simulink model "Aerogen2019NoActuator"  (R2019b)
settings: Solver=FixedStepAuto  StartTime=0.0  StopTime=10  FixedStep=0.001  RelTol=1e-6  EnableMultiTasking=on
values from neighbouring files (symbols this model uses):
  Bm = 0.001    [Trim_Lin.m]    (also in controlExercise.m)
  c1 = 0.51763    [Trim_Lin.m]    (also in controlExercise.m)
  c2 = 116    [Trim_Lin.m]    (also in controlExercise.m)
  c3 = 0.4    [Trim_Lin.m]    (also in controlExercise.m)
  c4 = 5    [Trim_Lin.m]    (also in controlExercise.m)
  c5 = 21    [Trim_Lin.m]    (also in controlExercise.m)
  c6 = 0.006795    [Trim_Lin.m]    (also in controlExercise.m)
  J = 10    [Trim_Lin.m]    (also in controlExercise.m = 0.1)
  Ke = 1.3717    [Trim_Lin.m]    (also in controlExercise.m)
  La = 0.028    [Trim_Lin.m]    (also in controlExercise.m)
  R = 10    [Trim_Lin.m]    (also in controlExercise.m)
  Ra = 2.58    [Trim_Lin.m]    (also in controlExercise.m)
  Rho = 1.225    [Trim_Lin.m]    (also in controlExercise.m)
  Rpala = 1.6    [Trim_Lin.m]    (also in controlExercise.m)
  Tf = 0.1    [Trim_Lin.m]    (also in controlExercise.m)
  Vw = 10    [Trim_Lin.m]    (also in controlExercise.m)
settings Model: ExtModeTrigDuration=100  Creator=Ignacio  LastModifiedBy=Carlos
settings SolverCC: PositivePriorityOrder=on
settings DataIOCC: LimitDataPoints=on  SaveFormat=Array  ReturnWorkspaceOutputs=off
settings OptimizationCC: DefaultParameterBehavior=Inlined  LifeSpan=1  MaxStackSize=64  EfficientTunableParamExpr=on
settings DebuggingCC: UnderspecifiedInitializationDetection=Classic  MergeDetectMultiDrivingBlocksExec=none  AllowSymbolicDim=off  SFUnexpectedBacktrackingDiag=warning  SFNoUnconditionalDefaultTransitionDiag=warning  SFExecutionAtInitializationDiag=none  ArithmeticOperatorsInVariantConditions=warning
settings HardwareCC: ProdBitPerPointer=32  ProdBitPerSizeT=32  ProdBitPerPtrDiffT=32  ProdLargestAtomicInteger=Long  ProdLargestAtomicFloat=Double  ProdWordSize=32  ProdHWDeviceType=ARM Compatible->ARM Cortex
settings ModelReferenceCC: PropagateSignalLabelsOutOfModel=off
settings SFSimCC: SimUseLocalCustomCode=off  MATLABDynamicMemAlloc=off  CustomCodeUndefinedFunction=UseInterfaceOnly
settings RTWCC: SystemTargetFile=ert.tlc  TemplateMakefile=ert_default_tmf  GenerateReport=on  RTWVerbose=off  RTWUseLocalCustomCode=off  Toolchain=GNU GCC Raspberry Pi  IncludeHyperlinkInReport=on  LaunchReport=on  GenerateTraceInfo=on  GenerateTraceReport=on  GenerateTraceReportSl=on  GenerateTraceReportSf=on  GenerateTraceReportEml=on
settings CodeAppCC: ForceParamTrailComments=on  IgnoreCustomStorageClasses=off  OperatorAnnotations=on  SimulinkDataObjDesc=on  SFDataObjDesc=on  MATLABFcnDesc=on  InsertBlockDesc=on  StateflowObjectComments=on  MATLABSourceComments=on
settings ERTTargetCC: MultiwordLength=2048  SupportVariableSizeSignals=on  ERTCustomFileTemplate=example_file_process.tlc
settings ConfigComp: CovMetricSettings=dw  CovHTMLOptions=-sRT=1 -aTS=1 -bRG=1 -bTC=1 -hTR=0 -nFC=0 -scm=1 -bcm=1 -xEv=0  CovHtmlReporting=on  CovSaveCumulativeToWorkspaceVar=on  CovSaveSingleToWorkspaceVar=on  CovExternalEMLEnable=off  CovSFcnEnable=off
settings SimscapeCC: SimscapeNormalizeSystem=off  SelectedTab=SimMechanics2G
settings ConfigurationSet: Description=SimMechanics 2G

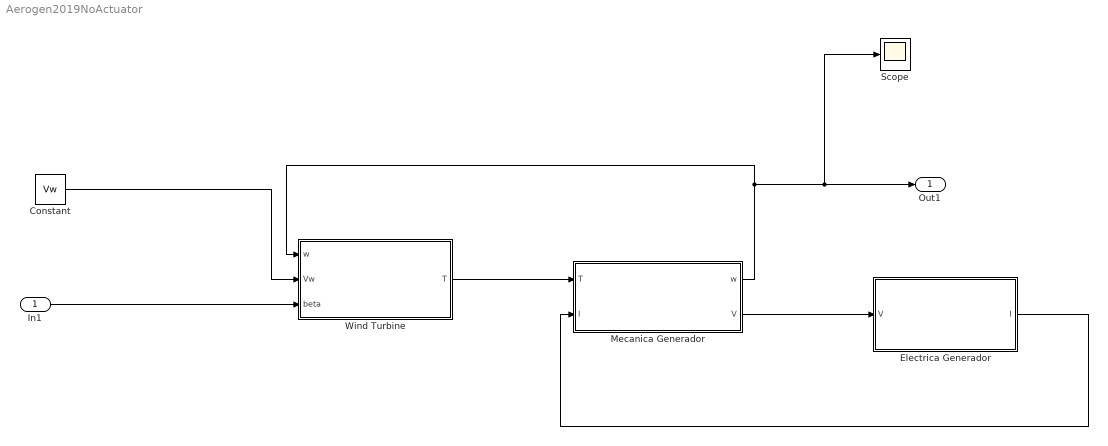
== system Aerogen2019NoActuator ==
  In1 : Inport
  Constant : Constant  Value=Vw
  Electrica Generador : Subsystem
  Mecanica Generador : Subsystem
  Scope : Scope
  Wind Turbine : Subsystem
  Out1 : Outport  VectorParamsAs1DForOutWhenUnconnected=off
  wires:
  Mecanica Generador/1(w) -> Wind Turbine/1(w), Scope/1, Out1/1
  Mecanica Generador/2(V) -> Electrica Generador/1(V)
  Electrica Generador/1(I) -> Mecanica Generador/2(I)
  Wind Turbine/1(T) -> Mecanica Generador/1(T)
  Constant/1 -> Wind Turbine/2(Vw)
  In1/1 -> Wind Turbine/3(beta)

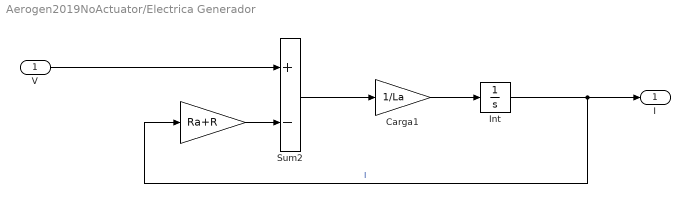
== system Aerogen2019NoActuator/Electrica Generador ==
  V : Inport
  " " : Gain  Gain=Ra+R
  Carga1 : Gain  Gain=1/La
  Int : Integrator
  Sum2 : Sum  Inputs=+-
  I : Outport  VectorParamsAs1DForOutWhenUnconnected=off
  wires:
  Int/1 -> " "/1, I/1  "I"
  Carga1/1 -> Int/1
  " "/1 -> Sum2/2
  V/1 -> Sum2/1
  Sum2/1 -> Carga1/1

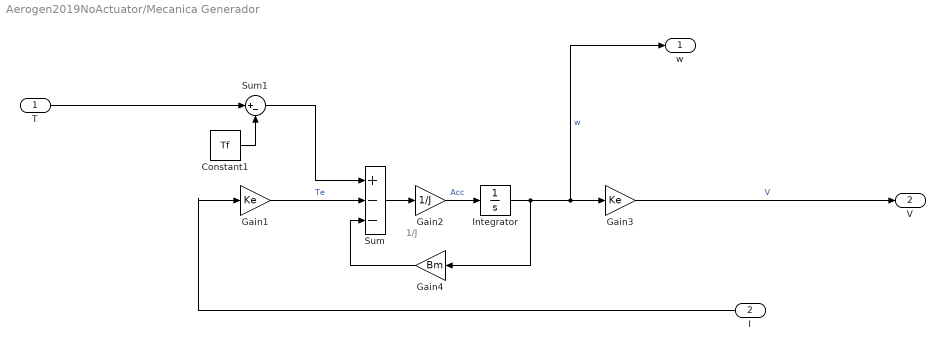
== system Aerogen2019NoActuator/Mecanica Generador ==
  note: 1/J
  T : Inport
  I : Inport  Port=2
  Constant1 : Constant  Value=Tf
  Gain1 : Gain  Gain=Ke  SaturateOnIntegerOverflow=on  OutDataTypeStr=Inherit: Same as input  ParamDataTypeStr=Inherit: Same as input
  Gain2 : Gain  Gain=1/J  SaturateOnIntegerOverflow=on  OutDataTypeStr=Inherit: Same as input  ParamDataTypeStr=Inherit: Same as input
  Gain3 : Gain  Gain=Ke  SaturateOnIntegerOverflow=on  OutDataTypeStr=Inherit: Same as input  ParamDataTypeStr=Inherit: Same as input
  Gain4 : Gain  Gain=Bm  SaturateOnIntegerOverflow=on  OutDataTypeStr=Inherit: Same as input  ParamDataTypeStr=Inherit: Same as input
  Integrator : Integrator  InitialCondition=1
  Sum : Sum  Inputs=+--  SaturateOnIntegerOverflow=on  InputSameDT=on  OutDataTypeStr=Inherit: Same as first input
  Sum1 : Sum  Inputs=|+-
  w : Outport  VectorParamsAs1DForOutWhenUnconnected=off
  V : Outport  Port=2  VectorParamsAs1DForOutWhenUnconnected=off
  wires:
  Constant1/1 -> Sum1/2
  Sum/1 -> Gain2/1
  I/1 -> Gain1/1
  Gain2/1 -> Integrator/1  "Acc"
  Gain1/1 -> Sum/2  "Te"
  Integrator/1 -> Gain4/1, w/1, Gain3/1  "w"
  Gain3/1 -> V/1  "V"
  T/1 -> Sum1/1
  Gain4/1 -> Sum/3
  Sum1/1 -> Sum/1

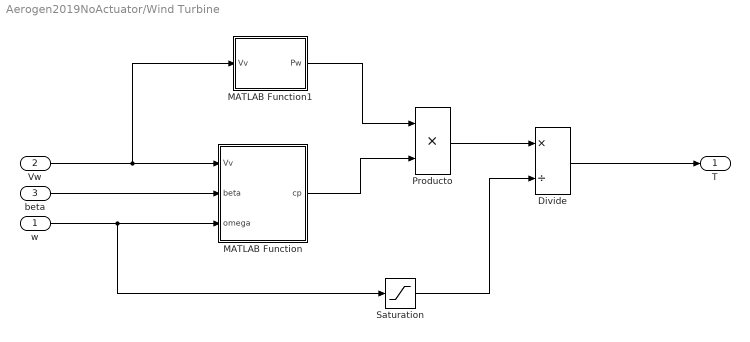
== system Aerogen2019NoActuator/Wind Turbine ==
  w : Inport
  Vw : Inport  Port=2
  beta : Inport  Port=3
  Divide : Product  Inputs=*/
  MATLAB Function : MATLAB Function  TreatAsAtomicUnit=on
  MATLAB Function1 : MATLAB Function  TreatAsAtomicUnit=on
  Producto : Product  Inputs=**
  Saturation : Saturate  UpperLimit=1000  LowerLimit=0.1
  T : Outport  VectorParamsAs1DForOutWhenUnconnected=off
  wires:
  beta/1 -> MATLAB Function/2(beta)
  Vw/1 -> MATLAB Function1/1(Vv), MATLAB Function/1(Vv)
  w/1 -> Saturation/1, MATLAB Function/3(omega)
  MATLAB Function1/1(Pw) -> Producto/1
  MATLAB Function/1(cp) -> Producto/2
  Producto/1 -> Divide/1
  Saturation/1 -> Divide/2
  Divide/1 -> T/1

== matlab function Aerogen2019NoActuator/Wind Turbine/MATLAB Function1 ==
  data: Vv input; Pw output; Rho parameter; Rpala parameter
function Pw = Pw(Vv,Rho,Rpala)
%#codegen

Pw=0.5*Rho*pi()*Rpala^2*Vv^3;

== matlab function Aerogen2019NoActuator/Wind Turbine/MATLAB Function ==
  data: Vv input; cp output; beta input; omega input; Rpala parameter; c1 parameter; c2 parameter; c3 parameter; c4 parameter; c5 parameter; c6 parameter
function cp = Cp(Vv,beta,omega,Rpala,c1,c2,c3,c4,c5,c6)
%#codegen
beta=-beta;
landa=omega*Rpala/Vv;
landai=1/(1/(landa+0.08*beta)-0.035/(1+beta^3));
cp=c1*(c2/landai-c3*beta-c4)*exp(-c5/landai)+c6*landa;
